simulink model "state_feedback_disturbance"  (R2016b)
settings: Solver=ode45  StartTime=0.0  StopTime=10.0  RelTol=1e-3
values from neighbouring files (symbols this model uses):
  C = [1 0 0 0 0;0 0 1 0 0]    [cee_SCRIPT.m]
  D = [0;0]    [cee_SCRIPT.m]
  K = lqr(A, B, Qr, Rr)    [cee_SCRIPT.m]
  T = 10    [cee_SCRIPT.m]
  x0c = deg2rad(x0c_graus)'    [cee_SCRIPT.m]
undefined symbols (not defined in the file or in its folder): A, B
libraries: simulink x2
settings Model: Creator=jmgri  LastModifiedBy=jmgri
settings OptimizationCC: LifeSpan=inf
settings DebuggingCC: SFExecutionAtInitializationDiag=none
settings HardwareCC: ProdBitPerSizeT=32  ProdBitPerPtrDiffT=32  ProdWordSize=32  ProdHWDeviceType=Specified

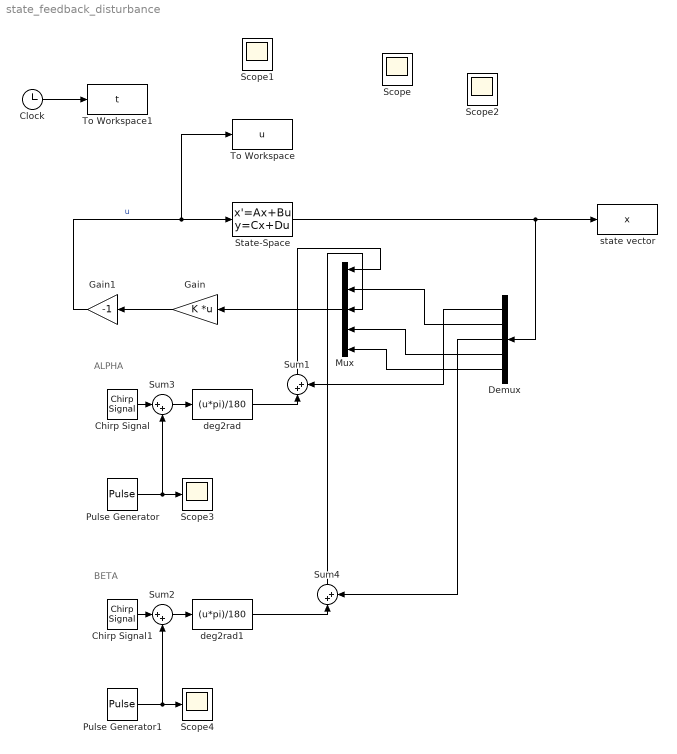
== system state_feedback_disturbance ==
  note: ALPHA
  note: BETA
  Chirp Signal : simulink/Sources/Chirp Signal  f1=0  T=T  f2=0
  Chirp Signal1 : simulink/Sources/Chirp Signal  f1=0  T=T  f2=0
  Clock : Clock
  Demux : Demux  Outputs=5
  Gain : Gain  Gain=K  Multiplication=Matrix(K*u)
  Gain1 : Gain  Gain=-1
  Mux : Mux  Inputs=5
  Pulse Generator : DiscretePulseGenerator  PulseType=Time based  Amplitude=0  Period=T  PulseWidth=70
  Pulse Generator1 : DiscretePulseGenerator  PulseType=Time based  Amplitude=0  Period=T  PulseWidth=70
  Scope{,1..4} (5 alike) : Scope
  State-Space : StateSpace  A=A  B=B  C=C  D=D  X0=x0c
  Sum{1..4} (4 alike) : Sum  Inputs=|++
  To Workspace : ToWorkspace  VariableName=u  SampleTime=-1
  To Workspace1 : ToWorkspace  VariableName=t  SampleTime=-1
  deg2rad : Fcn  Expr=(u*pi)/180
  deg2rad1 : Fcn  Expr=(u*pi)/180
  state vector : ToWorkspace  VariableName=x  SampleTime=-1
  wires:
  Gain/1 -> Gain1/1
  Gain1/1 -> To Workspace/1, State-Space/1  "u"
  State-Space/1 -> Demux/1, state vector/1
  Clock/1 -> To Workspace1/1
  Sum3/1 -> deg2rad/1
  Chirp Signal/1 -> Sum3/1
  Pulse Generator/1 -> Scope3/1, Sum3/2
  Mux/1 -> Gain/1
  deg2rad/1 -> Sum1/1
  Sum2/1 -> deg2rad1/1
  Chirp Signal1/1 -> Sum2/1
  Pulse Generator1/1 -> Scope4/1, Sum2/2
  deg2rad1/1 -> Sum4/1
  Demux/1 -> Sum1/2
  Sum1/1 -> Mux/1
  Demux/2 -> Mux/2
  Sum4/1 -> Mux/3
  Demux/3 -> Sum4/2
  Demux/4 -> Mux/4
  Demux/5 -> Mux/5
